simulink model "SEM_Battery"  (R2024a)
settings: Solver=FixedStepAuto  StartTime=0.0  StopTime=10.0  FixedStep=0.1  RelTol=1e-3
libraries: batteryecm_lib x96, fl_lib x4, nesl_utility x4, autolibmappedmotor x1
settings Model: Creator=v2578048  LastModifiedBy=marcelkaminski
settings RTWCC: GPUComputeCapability=3.5

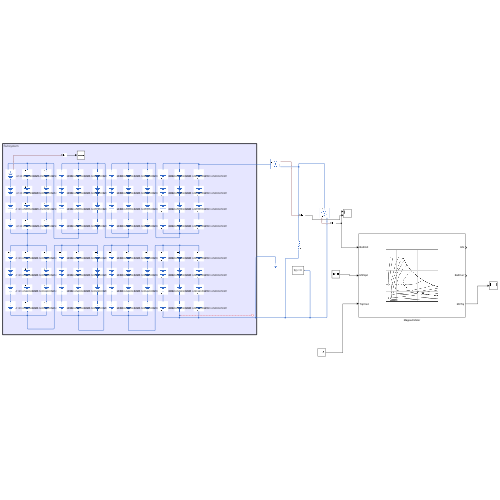
[thumbnail: Simulink's stored preview of the top-level diagram]
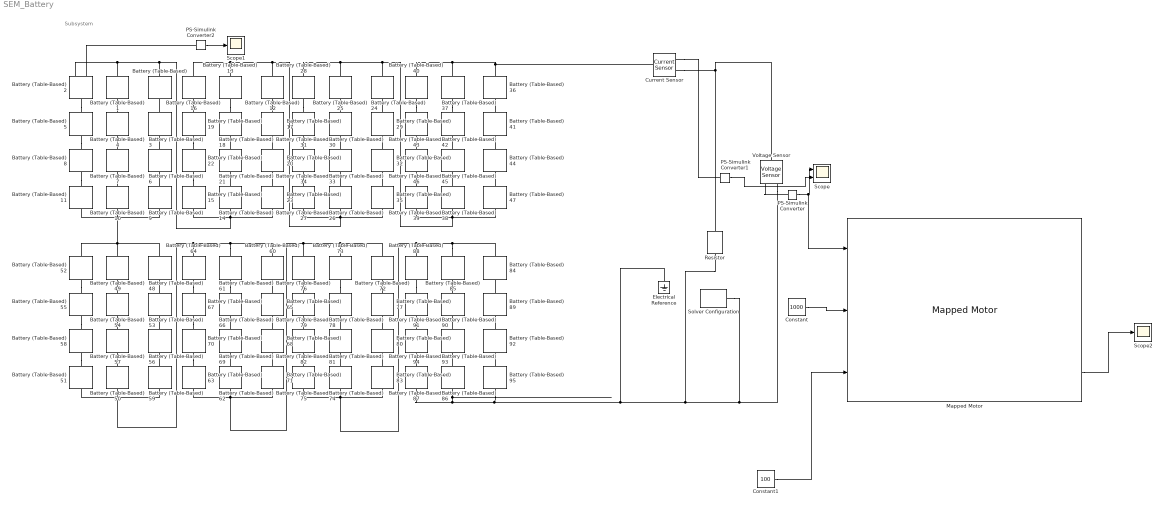
== system SEM_Battery ==
  note: Subsystem
  Battery (Table-Based){,1,3..95} (95 alike) : batteryecm_lib/Battery (Table-Based)  Tag={'toolbox/physmod/battery/shared_library/m/batteryecm_lib_parts';'Battery__Table_Based_/A123/ANR26650M1.xml'}  SOC_vec=[0 0.01 0.02 0.03 0.04 0.05 0.06 0.07 0.08 0.09 0.1 0.11 0.12 0.13 0.14 0.15 0.16 0.17 0.18 0.19 0.2 0.21 0.22 0.23 0.24 0.25 0.26 0.27 0.28 0.29 0.3 0.31 0.32 0.33 0.34 0.35 0.36 0.37 0.38 0.39 0.4 0.41 0.42 0.43 0.44 0.45 0.46 0.47 0.48 0.49 0.5 0.51 0.52 0.53 0.54 0.55 0.56 0.57 0.58 0.59 0.6 0.61 0.62 0.63 0.64 0.65 0.66 0.67 0.68 0.69 0.7 0.71 0.72 0.73 0.74 0.75 0.76 0.77 0.78 0.79 0.8 0.81 0.82 0.83 0.84 0.85 0.86 0.87 0.88 0.89 0.9 0.91 0.92 0.93 0.94 0.95 0.96 0.97 0.98 0.99 1]  T_dependence=simscape.enum.tablebattery.temperature_dependence.yes  prm_dir=simscape.enum.tablebattery.prm_dir.noCurrentDirectionality  T_vec=[-20 0 25] degC  V0_mat=[2.06518 2.06518 2.06518;2.68276 2.68276 2.68276;2.83127 2.83127 2.83127;2.93006 2.93006 2.93006;3.00018 3.00018 3.00018;3.05444 3.05444 3.05444;3.098 3.098 3.098;3.13677 3.13677 3.13677;3.17233 3.17233 3.17233;3.19687 3.19687 3.19687;3.20429 3.20429 3.20429;3.20797 3.20797 3.20797;3.21084 3.21084 3.21084;3.21322 3.21322 3.21322;3.21517 3.21517 3.21517;3.22057 3.22057 3.22057;3.22301 3.22301 3.22301;3.22946 3.22946 3.22946;3.23827 3.23827 3.23827;3.24173 3.24173 3.24173;3.24488 3.24488 3.24488;3.24931 3.24931 3.24931;3.2535 3.2535 3.2535;3.25765 3.25765 3.25765;3.26117 3.26117 3.26117;3.26357 3.26357 3.26357;3.26578 3.26578 3.26578;3.26981 3.26981 3.26981;3.27407 3.27407 3.27407;3.27754 3.27754 3.27754;3.27963 3.27963 3.27963;3.28165 3.28165 3.28165;3.28353 3.28353 3.28353;3.28542 3.28542 3.28542;3.28715 3.28715 3.28715;3.28889 3.28889 3.28889;3.29062 3.29062 3.29062;3.29275 3.29275 3.29275;3.29575 3.29575 3.29575;3.29889 3.29889 3.29889;3.30203 3.30203 3.30203;3.3027 3.3027 3.3027;3.30283 3.30283 3.30283;3.30242 3.30242 3.30242;3.30201 3.30201 3.30201;3.30226 3.30226 3.30226;3.30369 3.30369 3.30369;3.30511 3.30511 3.30511;3.3066 3.3066 3.3066;3.30845 3.30845 3.30845;3.30961 3.30961 3.30961;3.31045 3.31045 3.31045;3.31128 3.31128 3.31128;3.31212 3.31212 3.31212;3.31294 3.31294 3.31294;3.31336 3.31336 3.31336;3.31432 3.31432 3.31432;3.31596 3.31596 3.31596;3.3176 3.3176 3.3176;3.31906 3.31906 3.31906;3.32016 3.32016 3.32016;3.32147 3.32147 3.32147;3.32313 3.32313 3.32313;3.32479 3.32479 3.32479;3.32699 3.32699 3.32699;3.32924 3.32924 3.32924;3.33149 3.33149 3.33149;3.33281 3.33281 3.33281;3.33327 3.33327 3.33327;3.33363 3.33363 3.33363;3.33398 3.33398 3.33398;3.33434 3.33434 3.33434;3.33558 3.33558 3.33558;3.33748 3.33748 3.33748;3.33946 3.33946 3.33946;3.34145 3.34145 3.34145;3.34404 3.34404 3.34404;3.34672 3.34672 3.34672;3.34941 3.34941 3.34941;3.35026 3.35026 3.35026;3.35086 3.35086 3.35086;3.35091 3.35091 3.35091;3.35083 3.35083 3.35083;3.35192 3.35192 3.35192;3.35429 3.35429 3.35429;3.3566 3.3566 3.3566;3.35958 3.35958 3.35958;3.36218 3.36218 3.36218;3.36335 3.36335 3.36335;3.36552 3.36552 3.36552;3.36994 3.36994 3.36994;3.3722 3.3722 3.3722;3.3731 3.3731 3.3731;3.37515 3.37515 3.37515;3.37949 3.37949 3.37949;3.38971 3.38971 3.38971;3.40199 3.40199 3.40199;3.42645 3.42645 3.42645;3.48039 3.48039 3.48039;3.63268 3.63268 3.63268;3.84587 3.84587 3.84587] V  V0_vec=[2.06518 2.68276 2.83127 2.93006 3.00018 3.05444 3.098 3.13677 3.17233 3.19687 3.20429 3.20797 3.21084 3.21322 3.21517 3.22057 3.22301 3.22946 3.23827 3.24173 3.24488 3.24931 3.2535 3.25765 3.26117 3.26357 3.26578 3.26981 3.27407 3.27754 3.27963 3.28165 3.28353 3.28542 3.28715 3.28889 3.29062 3.29275 3.29575 3.29889 3.30203 3.3027 3.30283 3.30242 3.30201 3.30226 3.30369 3.30511 3.3066 3.30845 3.30961 3.31045 3.31128 3.31212 3.31294 3.31336 3.31432 3.31596 3.3176 3.31906 3.32016 3.32147 3.32313 3.32479 3.32699 3.32924 3.33149 3.33281 3.33327 3.33363 3.33398 3.33434 3.33558 3.33748 3.33946 3.34145 3.34404 3.34672 3.34941 3.35026 3.35086 3.35091 3.35083 3.35192 3.35429 3.3566 3.35958 3.36218 3.36335 3.36552 3.36994 3.3722 3.3731 3.37515 3.37949 3.38971 3.40199 3.42645 3.48039 3.63268 3.84587] V  V_range=[1.8 Inf] V  R0_mat=[0.28791 0.39917 0.03594;0.53384 0.62959 0.04836;0.57583 0.56865 0.04765;0.59621 0.50771 0.04556;0.60411 0.44678 0.04266;0.60512 0.38584 0.03932;0.60148 0.35318 0.03569;0.59575 0.33243 0.03191;0.58863 0.31331 0.02805;0.57672 0.29803 0.02388;0.55737 0.27565 0.02036;0.53639 0.25442 0.01833;0.51511 0.23302 0.01708;0.50085 0.21733 0.01587;0.48831 0.20337 0.01474;0.47733 0.19108 0.01411;0.46518 0.17861 0.01378;0.45492 0.16789 0.01359;0.44686 0.15933 0.01333;0.43712 0.15091 0.01312;0.42864 0.14235 0.01302;0.42073 0.13523 0.01308;0.41279 0.13112 0.01313;0.40493 0.127 0.01318;0.39734 0.12273 0.01323;0.38927 0.11936 0.01327;0.38209 0.11591 0.01333;0.37585 0.11324 0.01346;0.36956 0.11236 0.0136;0.36284 0.11117 0.01363;0.35652 0.10939 0.01363;0.35104 0.10772 0.01362;0.34554 0.10751 0.01361;0.34017 0.1073 0.01363;0.33473 0.10703 0.01368;0.32958 0.10675 0.01374;0.32594 0.10584 0.01379;0.32247 0.10427 0.01385;0.31911 0.10309 0.01395;0.31579 0.10197 0.01407;0.31253 0.1013 0.01419;0.30825 0.10101 0.01424;0.30375 0.10049 0.01428;0.29928 0.09973 0.01426;0.29512 0.09897 0.01424;0.29126 0.09851 0.01424;0.28925 0.09882 0.01427;0.28727 0.09919 0.01431;0.28531 0.09959 0.01435;0.2831 0.09941 0.01443;0.2802 0.09868 0.0145;0.27716 0.09781 0.01456;0.27412 0.09713 0.01462;0.26933 0.09664 0.01468;0.26437 0.09613 0.01473;0.26155 0.09545 0.01474;0.26216 0.09509 0.01476;0.26306 0.09503 0.0148;0.26159 0.09497 0.01484;0.25849 0.09478 0.01488;0.25493 0.09441 0.0149;0.25109 0.09413 0.01492;0.24864 0.09443 0.01498;0.24734 0.09474 0.01504;0.24628 0.09481 0.01513;0.24523 0.09489 0.01523;0.24431 0.09498 0.01532;0.24301 0.09496 0.01539;0.24134 0.09492 0.01543;0.23962 0.09482 0.01545;0.23798 0.09473 0.01547;0.23639 0.09464 0.0155;0.2352 0.09494 0.01554;0.23428 0.09522 0.01561;0.23339 0.09501 0.01566;0.23251 0.0948 0.01572;0.23188 0.09479 0.0158;0.23129 0.09474 0.01589;0.23109 0.09468 0.01598;0.2301 0.09394 0.01601;0.229 0.09311 0.01605;0.22766 0.09205 0.01609;0.22633 0.09165 0.01612;0.22553 0.09189 0.01613;0.22529 0.09268 0.01616;0.22504 0.09302 0.01619;0.22516 0.09346 0.01618;0.22512 0.09375 0.01594;0.22445 0.09333 0.0156;0.22379 0.09334 0.01534;0.22383 0.09429 0.01512;0.22294 0.09419 0.01474;0.22121 0.0935 0.01431;0.21784 0.09272 0.01395;0.21547 0.09199 0.01345;0.21296 0.09382 0.01301;0.20996 0.09444 0.01263;0.20584 0.09405 0.01235;0.21023 0.09408 0.01272;0.21135 0.10392 0.01483;0.19733 0.12789 0.01454] Ohm  R0_vec=[0.03594 0.04836 0.04765 0.04556 0.04266 0.03932 0.03569 0.03191 0.02805 0.02388 0.02036 0.01833 0.01708 0.01587 0.01474 0.01411 0.01378 0.01359 0.01333 0.01312 0.01302 0.01308 0.01313 0.01318 0.01323 0.01327 0.01333 0.01346 0.0136 0.01363 0.01363 0.01362 0.01361 0.01363 0.01368 0.01374 0.01379 0.01385 0.01395 0.01407 0.01419 0.01424 0.01428 0.01426 0.01424 0.01424 0.01427 0.01431 0.01435 0.01443 0.0145 0.01456 0.01462 0.01468 0.01473 0.01474 0.01476 0.0148 0.01484 0.01488 0.0149 0.01492 0.01498 0.01504 0.01513 0.01523 0.01532 0.01539 0.01543 0.01545 0.01547 0.0155 0.01554 0.01561 0.01566 0.01572 0.0158 0.01589 0.01598 0.01601 0.01605 0.01609 0.01612 0.01613 0.01616 0.01619 0.01618 0.01594 0.0156 0.01534 0.01512 0.01474 0.01431 0.01395 0.01345 0.01301 0.01263 0.01235 0.01272 0.01483 0.01454] Ohm  R0_dis_mat=[.0117, .0085, .009; .011, .0085, .009; .0114, .0087, .0092; .0107, .0082, .0088; .0107, .0083, .0091; .0113, .0085, .0089; .0116, .0085, .0089] % Parameter not set Ohm  R0_dis_vec=[.0085, .0085, .0087, .0082, .0083, .0085, .0085] % Parameter not set Ohm  R0_ch_mat=[.0117, .0085, .009; .011, .0085, .009; .0114, .0087, .0092; .0107, .0082, .0088; .0107, .0083, .0091; .0113, .0085, .0089; .0116, .0085, .0089] % Parameter not set Ohm  R0_ch_vec=[.0085, .0085, .0087, .0082, .0083, .0085, .0085] % Parameter not set Ohm  AH=2.341 hr*A  prm_leak=simscape.enum.tablebattery.prm_leak.disabled  Rleak_vec=[8000, 7000, 6000] % Parameter not set Ohm  Rleak=7e3 % Parameter not set Ohm  extrapolation_option=simscape.enum.extrapolation.nearest  SOC_port=simscape.enum.tablebattery.enable.no  prm_dyn=simscape.enum.tablebattery.prm_dyn.off  R1_mat=[.0109, .0029, .0013; .0069, .0024, .0012; .0047, .0026, .0013; .0034, .0016, .001; .0033, .0023, .0014; .0033, .0018, .0011; .0028, .0017, .0011] % Parameter not set Ohm  R1_vec=[.0029, .0024, .0026, .0016, .0023, .0018, .0017] % Parameter not set Ohm  tau1_mat=[20, 36, 39; 31, 45, 39; 109, 105, 61; 36, 29, 26; 59, 77, 67; 40, 33, 29; 25, 39, 33] % Parameter not set s  tau1_vec=[36, 45, 105, 29, 77, 33, 39] % Parameter not set s  R2_mat=[.0109, .0029, .0013; .0069, .0024, .0012; .0047, .0026, .0013; .0034, .0016, .001; .0033, .0023, .0014; .0033, .0018, .0011; .0028, .0017, .0011] % Parameter not set Ohm  R2_vec=[.0029, .0024, .0026, .0016, .0023, .0018, .0017] % Parameter not set Ohm  tau2_mat=[20, 36, 39; 31, 45, 39; 109, 105, 61; 36, 29, 26; 59, 77, 67; 40, 33, 29; 25, 39, 33] % Parameter not set s  tau2_vec=[36, 45, 105, 29, 77, 33, 39] % Parameter not set s  R3_mat=[.0109, .0029, .0013; .0069, .0024, .0012; .0047, .0026, .0013; .0034, .0016, .001; .0033, .0023, .0014; .0033, .0018, .0011; .0028, .0017, .0011] % Parameter not set Ohm  R3_vec=[.0029, .0024, .0026, .0016, .0023, .0018, .0017] % Parameter not set Ohm  tau3_mat=[20, 36, 39; 31, 45, 39; 109, 105, 61; 36, 29, 26; 59, 77, 67; 40, 33, 29; 25, 39, 33] % Parameter not set s  tau3_vec=[36, 45, 105, 29, 77, 33, 39] % Parameter not set s  R4_mat=[.0109, .0029, .0013; .0069, .0024, .0012; .0047, .0026, .0013; .0034, .0016, .001; .0033, .0023, .0014; .0033, .0018, .0011; .0028, .0017, .0011] % Parameter not set Ohm  R4_vec=[.0029, .0024, .0026, .0016, .0023, .0018, .0017] % Parameter not set Ohm  tau4_mat=[20, 36, 39; 31, 45, 39; 109, 105, 61; 36, 29, 26; 59, 77, 67; 40, 33, 29; 25, 39, 33] % Parameter not set s  tau4_vec=[36, 45, 105, 29, 77, 33, 39] % Parameter not set s  R5_mat=[.0109, .0029, .0013; .0069, .0024, .0012; .0047, .0026, .0013; .0034, .0016, .001; .0033, .0023, .0014; .0033, .0018, .0011; .0028, .0017, .0011] % Parameter not set Ohm  R5_vec=[.0029, .0024, .0026, .0016, .0023, .0018, .0017] % Parameter not set Ohm  tau5_mat=[20, 36, 39; 31, 45, 39; 109, 105, 61; 36, 29, 26; 59, 77, 67; 40, 33, 29; 25, 39, 33] % Parameter not set s  tau5_vec=[36, 45, 105, 29, 77, 33, 39] % Parameter not set s  prm_fade=simscape.enum.tablebattery.prm_fade.tableN  N0=100 % Parameter not set  dV0=0 % Parameter not set  dR0=0 % Parameter not set  dAH=0 % Parameter not set  dRleak=0 % Parameter not set  dR1=0 % Parameter not set  dR2=0 % Parameter not set  dR3=0 % Parameter not set  dR4=0 % Parameter not set  dR5=0 % Parameter not set  N0vec=[1 12 23 34 45 56 67 78 89 100 111 122 133 144 155 166 177 188 199 210 221 232 243 254 265 276 287 298 309 320 331 342 353 364 375 386 397 408 419 430 441 452 463 474 485 496 507 518 529 540 551 562 573 584 595 606 617 628 639 650 661 672 683 694 705 716 727 738 749 760 771 782 793 804 815 826 837 848 859 870 881 892 903 914 925 936 947 958 969 980 991 1002]  Tfadevec=[298.15, 323.15] % Parameter not set K  dV0vec=[0 -2.002 -2.6261 -2.9216 -3.1236 -3.3257 -3.5223 -3.7133 -3.9044 -4.2968 -4.7603 -5.2239 -5.6645 -6.0494 -6.4343 -6.8192 -7.2041 -7.3674 -7.2786 -7.1898 -7.101 -7.1198 -7.4721 -7.8245 -8.1769 -8.5292 -8.8816 -9.2733 -9.5616 -9.7015 -9.8414 -9.9678 -10.0299 -10.0919 -10.154 -10.216 -10.2781 -10.3402 -10.4448 -10.5636 -10.6824 -10.8012 -10.9056 -10.9361 -10.9667 -10.9972 -11.0226 -11.0377 -11.0527 -11.0678 -11.0979 -11.1585 -11.2191 -11.2797 -11.3402 -11.3884 -11.4143 -11.4403 -11.4662 -11.4921 -11.5332 -11.5611 -11.5848 -11.6085 -11.6323 -11.6445 -11.6495 -11.6545 -11.6594 -11.6644 -11.6693 -11.6918 -11.7308 -11.7699 -11.8089 -11.848 -11.8797 -11.8797 -11.8797 -11.8797 -11.8872 -11.8994 -11.9116 -11.9238 -11.9426 -11.968 -11.9934 -12.0155 -12.0345 -12.0535 -12.0755 -12.0979]  dR0vec=[0 0 0 0 0 0 0 0 0 0 0 0 0 0 0 0 0 0 0 0 0 0 0 0 0 0 0 0 0 0 0 0 0 0 0 0 0 0 0 0 0 0 0 0 0 0 0 0 0 0 0 0 0 0 0 0 0 0 0 0 0 0 0 0 0 0 0 0 0 0 0 0 0 0 0 0 0 0 0 0 0 0 0 0 0 0 0 0 0 0 0 0] % Parameter assumed  dAHvec=[0 -0.361 -0.474 -0.527 -0.564 -0.6 -0.635 -0.67 -0.704 -0.775 -0.859 -0.942 -1.031 -1.128 -1.225 -1.322 -1.419 -1.461 -1.438 -1.416 -1.393 -1.398 -1.487 -1.576 -1.665 -1.754 -1.843 -1.942 -2.042 -2.141 -2.241 -2.331 -2.376 -2.42 -2.464 -2.508 -2.553 -2.597 -2.671 -2.756 -2.841 -2.926 -3 -3.048 -3.096 -3.144 -3.184 -3.208 -3.231 -3.255 -3.302 -3.398 -3.493 -3.588 -3.683 -3.759 -3.8 -3.841 -3.881 -3.922 -3.987 -4.061 -4.135 -4.21 -4.284 -4.323 -4.338 -4.354 -4.369 -4.385 -4.4 -4.47 -4.593 -4.715 -4.837 -4.96 -5.071 -5.071 -5.071 -5.071 -5.099 -5.145 -5.191 -5.237 -5.307 -5.403 -5.499 -5.582 -5.653 -5.725 -5.807 -5.892]  dRleakvec=[0, 0, 0] % Parameter not set  dR1vec=[0, 0, 0] % Parameter not set  dR2vec=[0, 0, 0] % Parameter not set  dR3vec=[0, 0, 0] % Parameter not set  dR4vec=[0, 0, 0] % Parameter not set  dR5vec=[0, 0, 0] % Parameter not set  dV0mat=[0, 0; 0, 0; 0, 0] % Parameter not set  dR0mat=[0, 0; 0, 0; 0, 0] % Parameter not set  dAHmat=[0, 0; 0, 0; 0, 0] % Parameter not set  dRleakmat=[0, 0; 0, 0; 0, 0] % Parameter not set  dR1mat=[0, 0; 0, 0; 0, 0] % Parameter not set  dR2mat=[0, 0; 0, 0; 0, 0] % Parameter not set  dR3mat=[0, 0; 0, 0; 0, 0] % Parameter not set  dR4mat=[0, 0; 0, 0; 0, 0] % Parameter not set  dR5mat=[0, 0; 0, 0; 0, 0] % Parameter not set  prm_age_modeling=simscape.enum.tablebattery.prm_age_modeling.equation  storage_dt_age_vec=[0] % Parameter not set d  storage_T_age_vec=[273] % Parameter not set K  prm_age_OCV=simscape.enum.tablebattery.prm_age_OCV.OCV  OCV_age=0.9 % Parameter not set  SOC_age=0.6 % Parameter not set  prm_age_resistance=simscape.enum.tablebattery.prm_age.disabled  OCV_scaling_age_resistance=2.2134e6 % Parameter not set  OCV_offset_age_resistance=1.632e6 % Parameter not set  temp_exp_age_resistance=0.515833569 % Parameter not set V  t_exp_age_resistance=0.75 % Parameter not set  T_age_vec_resistance=[273.15, 298.15, 323.15] % Parameter not set K  dt_age_vec_resistance=[90, 180, 270, 360] % Parameter not set d  dR0_age_vec=[0, 0, 0] % Parameter not set  t_meas_dR0_age=100 % Parameter not set d  dR0_age_mat=[0, 0, 0; 0, 0, 0; 0, 0, 0; 0, 0, 0] % Parameter not set  prm_age_capacity=simscape.enum.tablebattery.prm_age.disabled  OCV_scaling_age_capacity=1.5097e07 % Parameter not set  OCV_offset_age_capacity=8.3625e06 % Parameter not set  temp_exp_age_capacity=0.6011 % Parameter not set V  t_exp_age_capacity=0.75 % Parameter not set  T_age_vec_capacity=[273.15, 298.15, 323.15] % Parameter not set K  dt_age_vec_capacity=[90, 180, 270, 360] % Parameter not set d  dAH_age_vec=[0, 0, 0] % Parameter not set  t_meas_dAH_age=100 % Parameter not set d  dAH_age_mat=[0, 0, 0; 0, 0, 0; 0, 0, 0; 0, 0, 0] % Parameter not set  thermal_port=simscape.enum.thermaleffects.omit  temperature=298.15 % Parameter not set K  thermal_mass=64.8 % Parameter assumed J/K  i_specify=off  i_priority=None  i=0 A  i_nominal_specify=off  i_nominal_value=1  i_nominal_unit=A  v_specify=off  v_priority=None  v=0 V  v_nominal_specify=off  v_nominal_value=1  v_nominal_unit=V  stateOfCharge_specify=off  stateOfCharge_priority=High  stateOfCharge=1  stateOfCharge_nominal_specify=off  stateOfCharge_nominal_value=1  stateOfCharge_nominal_unit=1  num_cycles_specify=off  num_cycles_priority=High  num_cycles=0  num_cycles_nominal_specify=off  num_cycles_nominal_value=1  num_cycles_nominal_unit=1  cell_temperature_specify=off  cell_temperature_priority=High  cell_temperature=298.15 K  cell_temperature_nominal_specify=off  cell_temperature_nominal_value=1  cell_temperature_nominal_unit=K
      settings: AttributesFormatString=A123:ANR26650M1  InternalSimscapePortConfiguration="{\"Bottom\":[],\"Left\":[{\"id\":\"p\",\"label\":\"+\",\"type\":\"foundation.electrical.electrical\"}],\"Right\":[{\"id\":\"n\",\"label\":\"-\",\"type\":\"foundation.electrical.electrical\"}],\"Top\":[]}"
      settings: LibrarySourceBlock=|
      | batt_lib/Cells/Battery
      | (Table-Based)
  Battery (Table-Based)2 : batteryecm_lib/Battery (Table-Based)  Tag={'toolbox/physmod/battery/shared_library/m/batteryecm_lib_parts';'Battery__Table_Based_/A123/ANR26650M1.xml'}  SOC_vec=[0 0.01 0.02 0.03 0.04 0.05 0.06 0.07 0.08 0.09 0.1 0.11 0.12 0.13 0.14 0.15 0.16 0.17 0.18 0.19 0.2 0.21 0.22 0.23 0.24 0.25 0.26 0.27 0.28 0.29 0.3 0.31 0.32 0.33 0.34 0.35 0.36 0.37 0.38 0.39 0.4 0.41 0.42 0.43 0.44 0.45 0.46 0.47 0.48 0.49 0.5 0.51 0.52 0.53 0.54 0.55 0.56 0.57 0.58 0.59 0.6 0.61 0.62 0.63 0.64 0.65 0.66 0.67 0.68 0.69 0.7 0.71 0.72 0.73 0.74 0.75 0.76 0.77 0.78 0.79 0.8 0.81 0.82 0.83 0.84 0.85 0.86 0.87 0.88 0.89 0.9 0.91 0.92 0.93 0.94 0.95 0.96 0.97 0.98 0.99 1]  T_dependence=simscape.enum.tablebattery.temperature_dependence.yes  prm_dir=simscape.enum.tablebattery.prm_dir.noCurrentDirectionality  T_vec=[-20 0 25] degC  V0_mat=[2.06518 2.06518 2.06518;2.68276 2.68276 2.68276;2.83127 2.83127 2.83127;2.93006 2.93006 2.93006;3.00018 3.00018 3.00018;3.05444 3.05444 3.05444;3.098 3.098 3.098;3.13677 3.13677 3.13677;3.17233 3.17233 3.17233;3.19687 3.19687 3.19687;3.20429 3.20429 3.20429;3.20797 3.20797 3.20797;3.21084 3.21084 3.21084;3.21322 3.21322 3.21322;3.21517 3.21517 3.21517;3.22057 3.22057 3.22057;3.22301 3.22301 3.22301;3.22946 3.22946 3.22946;3.23827 3.23827 3.23827;3.24173 3.24173 3.24173;3.24488 3.24488 3.24488;3.24931 3.24931 3.24931;3.2535 3.2535 3.2535;3.25765 3.25765 3.25765;3.26117 3.26117 3.26117;3.26357 3.26357 3.26357;3.26578 3.26578 3.26578;3.26981 3.26981 3.26981;3.27407 3.27407 3.27407;3.27754 3.27754 3.27754;3.27963 3.27963 3.27963;3.28165 3.28165 3.28165;3.28353 3.28353 3.28353;3.28542 3.28542 3.28542;3.28715 3.28715 3.28715;3.28889 3.28889 3.28889;3.29062 3.29062 3.29062;3.29275 3.29275 3.29275;3.29575 3.29575 3.29575;3.29889 3.29889 3.29889;3.30203 3.30203 3.30203;3.3027 3.3027 3.3027;3.30283 3.30283 3.30283;3.30242 3.30242 3.30242;3.30201 3.30201 3.30201;3.30226 3.30226 3.30226;3.30369 3.30369 3.30369;3.30511 3.30511 3.30511;3.3066 3.3066 3.3066;3.30845 3.30845 3.30845;3.30961 3.30961 3.30961;3.31045 3.31045 3.31045;3.31128 3.31128 3.31128;3.31212 3.31212 3.31212;3.31294 3.31294 3.31294;3.31336 3.31336 3.31336;3.31432 3.31432 3.31432;3.31596 3.31596 3.31596;3.3176 3.3176 3.3176;3.31906 3.31906 3.31906;3.32016 3.32016 3.32016;3.32147 3.32147 3.32147;3.32313 3.32313 3.32313;3.32479 3.32479 3.32479;3.32699 3.32699 3.32699;3.32924 3.32924 3.32924;3.33149 3.33149 3.33149;3.33281 3.33281 3.33281;3.33327 3.33327 3.33327;3.33363 3.33363 3.33363;3.33398 3.33398 3.33398;3.33434 3.33434 3.33434;3.33558 3.33558 3.33558;3.33748 3.33748 3.33748;3.33946 3.33946 3.33946;3.34145 3.34145 3.34145;3.34404 3.34404 3.34404;3.34672 3.34672 3.34672;3.34941 3.34941 3.34941;3.35026 3.35026 3.35026;3.35086 3.35086 3.35086;3.35091 3.35091 3.35091;3.35083 3.35083 3.35083;3.35192 3.35192 3.35192;3.35429 3.35429 3.35429;3.3566 3.3566 3.3566;3.35958 3.35958 3.35958;3.36218 3.36218 3.36218;3.36335 3.36335 3.36335;3.36552 3.36552 3.36552;3.36994 3.36994 3.36994;3.3722 3.3722 3.3722;3.3731 3.3731 3.3731;3.37515 3.37515 3.37515;3.37949 3.37949 3.37949;3.38971 3.38971 3.38971;3.40199 3.40199 3.40199;3.42645 3.42645 3.42645;3.48039 3.48039 3.48039;3.63268 3.63268 3.63268;3.84587 3.84587 3.84587] V  V0_vec=[2.06518 2.68276 2.83127 2.93006 3.00018 3.05444 3.098 3.13677 3.17233 3.19687 3.20429 3.20797 3.21084 3.21322 3.21517 3.22057 3.22301 3.22946 3.23827 3.24173 3.24488 3.24931 3.2535 3.25765 3.26117 3.26357 3.26578 3.26981 3.27407 3.27754 3.27963 3.28165 3.28353 3.28542 3.28715 3.28889 3.29062 3.29275 3.29575 3.29889 3.30203 3.3027 3.30283 3.30242 3.30201 3.30226 3.30369 3.30511 3.3066 3.30845 3.30961 3.31045 3.31128 3.31212 3.31294 3.31336 3.31432 3.31596 3.3176 3.31906 3.32016 3.32147 3.32313 3.32479 3.32699 3.32924 3.33149 3.33281 3.33327 3.33363 3.33398 3.33434 3.33558 3.33748 3.33946 3.34145 3.34404 3.34672 3.34941 3.35026 3.35086 3.35091 3.35083 3.35192 3.35429 3.3566 3.35958 3.36218 3.36335 3.36552 3.36994 3.3722 3.3731 3.37515 3.37949 3.38971 3.40199 3.42645 3.48039 3.63268 3.84587] V  V_range=[1.8 Inf] V  R0_mat=[0.28791 0.39917 0.03594;0.53384 0.62959 0.04836;0.57583 0.56865 0.04765;0.59621 0.50771 0.04556;0.60411 0.44678 0.04266;0.60512 0.38584 0.03932;0.60148 0.35318 0.03569;0.59575 0.33243 0.03191;0.58863 0.31331 0.02805;0.57672 0.29803 0.02388;0.55737 0.27565 0.02036;0.53639 0.25442 0.01833;0.51511 0.23302 0.01708;0.50085 0.21733 0.01587;0.48831 0.20337 0.01474;0.47733 0.19108 0.01411;0.46518 0.17861 0.01378;0.45492 0.16789 0.01359;0.44686 0.15933 0.01333;0.43712 0.15091 0.01312;0.42864 0.14235 0.01302;0.42073 0.13523 0.01308;0.41279 0.13112 0.01313;0.40493 0.127 0.01318;0.39734 0.12273 0.01323;0.38927 0.11936 0.01327;0.38209 0.11591 0.01333;0.37585 0.11324 0.01346;0.36956 0.11236 0.0136;0.36284 0.11117 0.01363;0.35652 0.10939 0.01363;0.35104 0.10772 0.01362;0.34554 0.10751 0.01361;0.34017 0.1073 0.01363;0.33473 0.10703 0.01368;0.32958 0.10675 0.01374;0.32594 0.10584 0.01379;0.32247 0.10427 0.01385;0.31911 0.10309 0.01395;0.31579 0.10197 0.01407;0.31253 0.1013 0.01419;0.30825 0.10101 0.01424;0.30375 0.10049 0.01428;0.29928 0.09973 0.01426;0.29512 0.09897 0.01424;0.29126 0.09851 0.01424;0.28925 0.09882 0.01427;0.28727 0.09919 0.01431;0.28531 0.09959 0.01435;0.2831 0.09941 0.01443;0.2802 0.09868 0.0145;0.27716 0.09781 0.01456;0.27412 0.09713 0.01462;0.26933 0.09664 0.01468;0.26437 0.09613 0.01473;0.26155 0.09545 0.01474;0.26216 0.09509 0.01476;0.26306 0.09503 0.0148;0.26159 0.09497 0.01484;0.25849 0.09478 0.01488;0.25493 0.09441 0.0149;0.25109 0.09413 0.01492;0.24864 0.09443 0.01498;0.24734 0.09474 0.01504;0.24628 0.09481 0.01513;0.24523 0.09489 0.01523;0.24431 0.09498 0.01532;0.24301 0.09496 0.01539;0.24134 0.09492 0.01543;0.23962 0.09482 0.01545;0.23798 0.09473 0.01547;0.23639 0.09464 0.0155;0.2352 0.09494 0.01554;0.23428 0.09522 0.01561;0.23339 0.09501 0.01566;0.23251 0.0948 0.01572;0.23188 0.09479 0.0158;0.23129 0.09474 0.01589;0.23109 0.09468 0.01598;0.2301 0.09394 0.01601;0.229 0.09311 0.01605;0.22766 0.09205 0.01609;0.22633 0.09165 0.01612;0.22553 0.09189 0.01613;0.22529 0.09268 0.01616;0.22504 0.09302 0.01619;0.22516 0.09346 0.01618;0.22512 0.09375 0.01594;0.22445 0.09333 0.0156;0.22379 0.09334 0.01534;0.22383 0.09429 0.01512;0.22294 0.09419 0.01474;0.22121 0.0935 0.01431;0.21784 0.09272 0.01395;0.21547 0.09199 0.01345;0.21296 0.09382 0.01301;0.20996 0.09444 0.01263;0.20584 0.09405 0.01235;0.21023 0.09408 0.01272;0.21135 0.10392 0.01483;0.19733 0.12789 0.01454] Ohm  R0_vec=[0.03594 0.04836 0.04765 0.04556 0.04266 0.03932 0.03569 0.03191 0.02805 0.02388 0.02036 0.01833 0.01708 0.01587 0.01474 0.01411 0.01378 0.01359 0.01333 0.01312 0.01302 0.01308 0.01313 0.01318 0.01323 0.01327 0.01333 0.01346 0.0136 0.01363 0.01363 0.01362 0.01361 0.01363 0.01368 0.01374 0.01379 0.01385 0.01395 0.01407 0.01419 0.01424 0.01428 0.01426 0.01424 0.01424 0.01427 0.01431 0.01435 0.01443 0.0145 0.01456 0.01462 0.01468 0.01473 0.01474 0.01476 0.0148 0.01484 0.01488 0.0149 0.01492 0.01498 0.01504 0.01513 0.01523 0.01532 0.01539 0.01543 0.01545 0.01547 0.0155 0.01554 0.01561 0.01566 0.01572 0.0158 0.01589 0.01598 0.01601 0.01605 0.01609 0.01612 0.01613 0.01616 0.01619 0.01618 0.01594 0.0156 0.01534 0.01512 0.01474 0.01431 0.01395 0.01345 0.01301 0.01263 0.01235 0.01272 0.01483 0.01454] Ohm  R0_dis_mat=[.0117, .0085, .009; .011, .0085, .009; .0114, .0087, .0092; .0107, .0082, .0088; .0107, .0083, .0091; .0113, .0085, .0089; .0116, .0085, .0089] % Parameter not set Ohm  R0_dis_vec=[.0085, .0085, .0087, .0082, .0083, .0085, .0085] % Parameter not set Ohm  R0_ch_mat=[.0117, .0085, .009; .011, .0085, .009; .0114, .0087, .0092; .0107, .0082, .0088; .0107, .0083, .0091; .0113, .0085, .0089; .0116, .0085, .0089] % Parameter not set Ohm  R0_ch_vec=[.0085, .0085, .0087, .0082, .0083, .0085, .0085] % Parameter not set Ohm  AH=2.341 hr*A  prm_leak=simscape.enum.tablebattery.prm_leak.disabled  Rleak_vec=[8000, 7000, 6000] % Parameter not set Ohm  Rleak=7e3 % Parameter not set Ohm  extrapolation_option=simscape.enum.extrapolation.nearest  SOC_port=simscape.enum.tablebattery.enable.yes  prm_dyn=simscape.enum.tablebattery.prm_dyn.off  R1_mat=[.0109, .0029, .0013; .0069, .0024, .0012; .0047, .0026, .0013; .0034, .0016, .001; .0033, .0023, .0014; .0033, .0018, .0011; .0028, .0017, .0011] % Parameter not set Ohm  R1_vec=[.0029, .0024, .0026, .0016, .0023, .0018, .0017] % Parameter not set Ohm  tau1_mat=[20, 36, 39; 31, 45, 39; 109, 105, 61; 36, 29, 26; 59, 77, 67; 40, 33, 29; 25, 39, 33] % Parameter not set s  tau1_vec=[36, 45, 105, 29, 77, 33, 39] % Parameter not set s  R2_mat=[.0109, .0029, .0013; .0069, .0024, .0012; .0047, .0026, .0013; .0034, .0016, .001; .0033, .0023, .0014; .0033, .0018, .0011; .0028, .0017, .0011] % Parameter not set Ohm  R2_vec=[.0029, .0024, .0026, .0016, .0023, .0018, .0017] % Parameter not set Ohm  tau2_mat=[20, 36, 39; 31, 45, 39; 109, 105, 61; 36, 29, 26; 59, 77, 67; 40, 33, 29; 25, 39, 33] % Parameter not set s  tau2_vec=[36, 45, 105, 29, 77, 33, 39] % Parameter not set s  R3_mat=[.0109, .0029, .0013; .0069, .0024, .0012; .0047, .0026, .0013; .0034, .0016, .001; .0033, .0023, .0014; .0033, .0018, .0011; .0028, .0017, .0011] % Parameter not set Ohm  R3_vec=[.0029, .0024, .0026, .0016, .0023, .0018, .0017] % Parameter not set Ohm  tau3_mat=[20, 36, 39; 31, 45, 39; 109, 105, 61; 36, 29, 26; 59, 77, 67; 40, 33, 29; 25, 39, 33] % Parameter not set s  tau3_vec=[36, 45, 105, 29, 77, 33, 39] % Parameter not set s  R4_mat=[.0109, .0029, .0013; .0069, .0024, .0012; .0047, .0026, .0013; .0034, .0016, .001; .0033, .0023, .0014; .0033, .0018, .0011; .0028, .0017, .0011] % Parameter not set Ohm  R4_vec=[.0029, .0024, .0026, .0016, .0023, .0018, .0017] % Parameter not set Ohm  tau4_mat=[20, 36, 39; 31, 45, 39; 109, 105, 61; 36, 29, 26; 59, 77, 67; 40, 33, 29; 25, 39, 33] % Parameter not set s  tau4_vec=[36, 45, 105, 29, 77, 33, 39] % Parameter not set s  R5_mat=[.0109, .0029, .0013; .0069, .0024, .0012; .0047, .0026, .0013; .0034, .0016, .001; .0033, .0023, .0014; .0033, .0018, .0011; .0028, .0017, .0011] % Parameter not set Ohm  R5_vec=[.0029, .0024, .0026, .0016, .0023, .0018, .0017] % Parameter not set Ohm  tau5_mat=[20, 36, 39; 31, 45, 39; 109, 105, 61; 36, 29, 26; 59, 77, 67; 40, 33, 29; 25, 39, 33] % Parameter not set s  tau5_vec=[36, 45, 105, 29, 77, 33, 39] % Parameter not set s  prm_fade=simscape.enum.tablebattery.prm_fade.tableN  N0=100 % Parameter not set  dV0=0 % Parameter not set  dR0=0 % Parameter not set  dAH=0 % Parameter not set  dRleak=0 % Parameter not set  dR1=0 % Parameter not set  dR2=0 % Parameter not set  dR3=0 % Parameter not set  dR4=0 % Parameter not set  dR5=0 % Parameter not set  N0vec=[1 12 23 34 45 56 67 78 89 100 111 122 133 144 155 166 177 188 199 210 221 232 243 254 265 276 287 298 309 320 331 342 353 364 375 386 397 408 419 430 441 452 463 474 485 496 507 518 529 540 551 562 573 584 595 606 617 628 639 650 661 672 683 694 705 716 727 738 749 760 771 782 793 804 815 826 837 848 859 870 881 892 903 914 925 936 947 958 969 980 991 1002]  Tfadevec=[298.15, 323.15] % Parameter not set K  dV0vec=[0 -2.002 -2.6261 -2.9216 -3.1236 -3.3257 -3.5223 -3.7133 -3.9044 -4.2968 -4.7603 -5.2239 -5.6645 -6.0494 -6.4343 -6.8192 -7.2041 -7.3674 -7.2786 -7.1898 -7.101 -7.1198 -7.4721 -7.8245 -8.1769 -8.5292 -8.8816 -9.2733 -9.5616 -9.7015 -9.8414 -9.9678 -10.0299 -10.0919 -10.154 -10.216 -10.2781 -10.3402 -10.4448 -10.5636 -10.6824 -10.8012 -10.9056 -10.9361 -10.9667 -10.9972 -11.0226 -11.0377 -11.0527 -11.0678 -11.0979 -11.1585 -11.2191 -11.2797 -11.3402 -11.3884 -11.4143 -11.4403 -11.4662 -11.4921 -11.5332 -11.5611 -11.5848 -11.6085 -11.6323 -11.6445 -11.6495 -11.6545 -11.6594 -11.6644 -11.6693 -11.6918 -11.7308 -11.7699 -11.8089 -11.848 -11.8797 -11.8797 -11.8797 -11.8797 -11.8872 -11.8994 -11.9116 -11.9238 -11.9426 -11.968 -11.9934 -12.0155 -12.0345 -12.0535 -12.0755 -12.0979]  dR0vec=[0 0 0 0 0 0 0 0 0 0 0 0 0 0 0 0 0 0 0 0 0 0 0 0 0 0 0 0 0 0 0 0 0 0 0 0 0 0 0 0 0 0 0 0 0 0 0 0 0 0 0 0 0 0 0 0 0 0 0 0 0 0 0 0 0 0 0 0 0 0 0 0 0 0 0 0 0 0 0 0 0 0 0 0 0 0 0 0 0 0 0 0] % Parameter assumed  dAHvec=[0 -0.361 -0.474 -0.527 -0.564 -0.6 -0.635 -0.67 -0.704 -0.775 -0.859 -0.942 -1.031 -1.128 -1.225 -1.322 -1.419 -1.461 -1.438 -1.416 -1.393 -1.398 -1.487 -1.576 -1.665 -1.754 -1.843 -1.942 -2.042 -2.141 -2.241 -2.331 -2.376 -2.42 -2.464 -2.508 -2.553 -2.597 -2.671 -2.756 -2.841 -2.926 -3 -3.048 -3.096 -3.144 -3.184 -3.208 -3.231 -3.255 -3.302 -3.398 -3.493 -3.588 -3.683 -3.759 -3.8 -3.841 -3.881 -3.922 -3.987 -4.061 -4.135 -4.21 -4.284 -4.323 -4.338 -4.354 -4.369 -4.385 -4.4 -4.47 -4.593 -4.715 -4.837 -4.96 -5.071 -5.071 -5.071 -5.071 -5.099 -5.145 -5.191 -5.237 -5.307 -5.403 -5.499 -5.582 -5.653 -5.725 -5.807 -5.892]  dRleakvec=[0, 0, 0] % Parameter not set  dR1vec=[0, 0, 0] % Parameter not set  dR2vec=[0, 0, 0] % Parameter not set  dR3vec=[0, 0, 0] % Parameter not set  dR4vec=[0, 0, 0] % Parameter not set  dR5vec=[0, 0, 0] % Parameter not set  dV0mat=[0, 0; 0, 0; 0, 0] % Parameter not set  dR0mat=[0, 0; 0, 0; 0, 0] % Parameter not set  dAHmat=[0, 0; 0, 0; 0, 0] % Parameter not set  dRleakmat=[0, 0; 0, 0; 0, 0] % Parameter not set  dR1mat=[0, 0; 0, 0; 0, 0] % Parameter not set  dR2mat=[0, 0; 0, 0; 0, 0] % Parameter not set  dR3mat=[0, 0; 0, 0; 0, 0] % Parameter not set  dR4mat=[0, 0; 0, 0; 0, 0] % Parameter not set  dR5mat=[0, 0; 0, 0; 0, 0] % Parameter not set  prm_age_modeling=simscape.enum.tablebattery.prm_age_modeling.equation  storage_dt_age_vec=[0] % Parameter not set d  storage_T_age_vec=[273] % Parameter not set K  prm_age_OCV=simscape.enum.tablebattery.prm_age_OCV.OCV  OCV_age=0.9 % Parameter not set  SOC_age=0.6 % Parameter not set  prm_age_resistance=simscape.enum.tablebattery.prm_age.disabled  OCV_scaling_age_resistance=2.2134e6 % Parameter not set  OCV_offset_age_resistance=1.632e6 % Parameter not set  temp_exp_age_resistance=0.515833569 % Parameter not set V  t_exp_age_resistance=0.75 % Parameter not set  T_age_vec_resistance=[273.15, 298.15, 323.15] % Parameter not set K  dt_age_vec_resistance=[90, 180, 270, 360] % Parameter not set d  dR0_age_vec=[0, 0, 0] % Parameter not set  t_meas_dR0_age=100 % Parameter not set d  dR0_age_mat=[0, 0, 0; 0, 0, 0; 0, 0, 0; 0, 0, 0] % Parameter not set  prm_age_capacity=simscape.enum.tablebattery.prm_age.disabled  OCV_scaling_age_capacity=1.5097e07 % Parameter not set  OCV_offset_age_capacity=8.3625e06 % Parameter not set  temp_exp_age_capacity=0.6011 % Parameter not set V  t_exp_age_capacity=0.75 % Parameter not set  T_age_vec_capacity=[273.15, 298.15, 323.15] % Parameter not set K  dt_age_vec_capacity=[90, 180, 270, 360] % Parameter not set d  dAH_age_vec=[0, 0, 0] % Parameter not set  t_meas_dAH_age=100 % Parameter not set d  dAH_age_mat=[0, 0, 0; 0, 0, 0; 0, 0, 0; 0, 0, 0] % Parameter not set  thermal_port=simscape.enum.thermaleffects.omit  temperature=298.15 % Parameter not set K  thermal_mass=64.8 % Parameter assumed J/K  i_specify=off  i_priority=None  i=0 A  i_nominal_specify=off  i_nominal_value=1  i_nominal_unit=A  v_specify=off  v_priority=None  v=0 V  v_nominal_specify=off  v_nominal_value=1  v_nominal_unit=V  stateOfCharge_specify=off  stateOfCharge_priority=High  stateOfCharge=1  stateOfCharge_nominal_specify=off  stateOfCharge_nominal_value=1  stateOfCharge_nominal_unit=1  num_cycles_specify=off  num_cycles_priority=High  num_cycles=0  num_cycles_nominal_specify=off  num_cycles_nominal_value=1  num_cycles_nominal_unit=1  cell_temperature_specify=off  cell_temperature_priority=High  cell_temperature=298.15 K  cell_temperature_nominal_specify=off  cell_temperature_nominal_value=1  cell_temperature_nominal_unit=K
      settings: AttributesFormatString=A123:ANR26650M1  InternalSimscapePortConfiguration="{\"Bottom\":[],\"Left\":[{\"id\":\"p\",\"label\":\"+\",\"type\":\"foundation.electrical.electrical\"},{\"id\":\"soc\",\"label\":\"SOC\",\"type\":\"output\"}],\"Right\":[{\"id\":\"n\",\"label\":\"-\",\"type\":\"foundation.electrical.electrical\"}],\"Top\":[]}"
      settings: LibrarySourceBlock=|
      | batt_lib/Cells/Battery
      | (Table-Based)
  Constant : Constant  Value=1000
  Constant1 : Constant  Value=100
  Current Sensor : fl_lib/Electrical/Electrical Sensors/Current Sensor
  Electrical Reference : fl_lib/Electrical/Electrical Elements/Electrical Reference
  Mapped Motor : autolibmappedmotor/Mapped Motor  port_config=Speed  param_by=Tabulated torque-speed envelope  w_t=[ 0 375 750 800 ]  T_t=[0.09 0.08 0.07 0]  torque_max=.1  power_max=30  Tc=0.02  param_loss=Single efficiency measurement  eff=100  w_eff=375  T_eff=0.08  Piron=0  Pbase=0  w_eff_bp=[-800 -400 0 400 800]  T_eff_bp=[0 0.03 0.06 0.09]  Temp_eff_bp=[233.15 293.15 373.15]  losses_table=[1.49 1.67 2.21 3.10; 0.42 0.69 1.14 2.03; 0.06 0.24 0.78 1.68; 0.42 0.69 1.14 2.03; 1.49 1.67 2.21 3.10]  losses_table_3d=cat(3,[1.49 1.67 2.21 3.10; 0.42 0.69 1.14 2.03; 0.06 0.24 0.78 1.68; 0.42 0.69 1.14 2.03; 1.49 1.67 2.21 3.10],[1.49 1.67 2.21 3.10; 0.42 0.69 1.14 2.03; 0.06 0.24 0.78 1.68; 0.42 0.69 1.14 2.03; 1.49 1.67 2.21 3.10],[1.49 1.67 2.21 3.10; 0.42 0.69 1.14 2.03; 0.06 0.24 0.78 1.68; 0.42 0.69 1.14 2.03; 1.49 1.67 2.21 3.10])  efficiency_table=[95 95 95 95; 95 95 95 95; 95 95 95 95; 95 95 95 95; 95 95 95 95]  efficiency_table_3d=cat(3,[95 95 95 95; 95 95 95 95; 95 95 95 95; 95 95 95 95; 95 95 95 95],[95 95 95 95; 95 95 95 95; 95 95 95 95; 95 95 95 95; 95 95 95 95],[95 95 95 95; 95 95 95 95; 95 95 95 95; 95 95 95 95; 95 95 95 95])  J=5e-6  b=1e-5  omega_o=0  T_t_extended=[0 0.07 0.08 0.09 0.08 0.07 0]  w_t_extended=[-800 -750 -375 0 375 750 800]  KLossIron=0  KLossCopper=0  x_w_eff_vec=[-8000 -4000 0 4000 8000]  x_T_eff_vec=[-0.09 -0.06 -0.03 0 0.03 0.06 0.09]  x_tmp_eff_vec=[-0.09 -0.06 -0.03 0 0.03 0.06 0.09]  x_losses_mat=[3.1 2.21 1.67 1.49 1.67 2.21 3.1;2.03 1.14 0.69 0.42 0.69 1.14 2.03;1.68 0.78 0.24 0.06 0.24 0.78 1.68;2.03 1.14 0.69 0.42 0.69 1.14 2.03;3.1 2.21 1.67 1.49 1.67 2.21 3.1]  x_losses_mat_3d=[37.8947368421052 25.2631578947368 12.6315789473684 0 12 24 36;18.9473684210526 12.6315789473684 6.3157894736842 0 5.99999999999999 12 18;0 0 0 0 0 0 0;18 12 5.99999999999999 0 6.3157894736842 12.6315789473684 18.9473684210526;36 24 12 0 12.6315789473684 25.2631578947368 37.8947368421052]  CalLossMapData={}  CalLossWithTempMapData={}  aMode=1  RefBlkName='autolibmappedmotor/Mapped Motor'
      settings: LibrarySourceBlock=autolibemachines/Mapped Motor
  PS-Simulink Converter : nesl_utility/PS-Simulink Converter  PhysicalDomain=network_engine_domain  SubClassName=ps_output  LeftPortType=input  RightPortType=output  PseudoPeriodic=off  Frequencies=[]  VectorFormat=inherit  Unit=inherit  AffineConversion=off
  PS-Simulink Converter1 : nesl_utility/PS-Simulink Converter  PhysicalDomain=network_engine_domain  SubClassName=ps_output  LeftPortType=input  RightPortType=output  PseudoPeriodic=off  Frequencies=[]  VectorFormat=inherit  Unit=inherit  AffineConversion=off
  PS-Simulink Converter2 : nesl_utility/PS-Simulink Converter  PhysicalDomain=network_engine_domain  SubClassName=ps_output  LeftPortType=input  RightPortType=output  PseudoPeriodic=off  Frequencies=[]  VectorFormat=inherit  Unit=inherit  AffineConversion=off
  Resistor : fl_lib/Electrical/Electrical Elements/Resistor  R=1 Ohm  i_specify=off  i_priority=None  i=0 A  i_nominal_specify=off  i_nominal_value=1  i_nominal_unit=A  v_specify=off  v_priority=None  v=0 V  v_nominal_specify=off  v_nominal_value=1  v_nominal_unit=V
  Scope : Scope  NumInputPorts=2
  Scope1 : Scope
  Scope2 : Scope
  Solver Configuration : nesl_utility/Solver Configuration  PhysicalDomain=network_engine_domain  SubClassName=solver  LeftPortType=input  RightPortType=generic  Tones=[]  Harmonics=[]  SimulateNoise=off  Profile=off  UseLocalSampling=off  EnableSwitchedLinearOptims=on  FrequencyDomain=off  UseCCode=off  RelTol=0.001  AbsTol=0.001  MinStep=1e-09  ToWorkspace=off  RevertToSquareIcSolve=off  NumHomotopyIterations=100  PhasorMode=off  PhasorModeNumHarmonics=1  ConsistencySolver=NEWTON_XTOL_AFTER_FTOL  IndexReductionMethod=DerivativeReplacement  DoDC=off  ResidualTolerance=1e-09  ConsistencyTolSource=GLOBAL  ConsistencyAbsTol=0.001  ConsistencyRelTol=0.001  ConsistencyTolFactor=0.001  UseLocalSolver=off  LocalSolverChoice=NE_BACKWARD_EULER_ADVANCER  ResolveIndetEquations=on  FunctionEvalNumThread=1  LocalSolverSampleTime=0.001  DoFixedCost=off  MaxNonlinIter=3  MaxModeIter=2  ComputeImpulses=off  ImpulseIterations=2  LinearAlgebra=auto  LinearAlgebraNumThread=0  EquationFormulation=NE_TIME_EF  DelaysMemoryBudget=1024  AutomaticFiltering=on  FilteringTimeConstant=0.001  PartitionStorageMethod=AS_NEEDED  PartitionMemoryBudget=1024  PartitionMethod=ROBUST  MultibodyUseLocalSolver=off  MultibodyLocalSolverChoice=ODE1  MultibodyLocalSolverSampleTime=0.001
  Voltage Sensor : fl_lib/Electrical/Electrical Sensors/Voltage Sensor
  wires:
  PS-Simulink Converter/1 -> Mapped Motor/1, Scope/1
  PS-Simulink Converter1/1 -> Scope/2
  PS-Simulink Converter2/1 -> Scope1/1
  Constant/1 -> Mapped Motor/2
  Constant1/1 -> Mapped Motor/3
  Mapped Motor/3 -> Scope2/1
  connections:
  PS-Simulink Converter/LConn1 -- Voltage Sensor/RConn1
  Current Sensor/RConn1 -- PS-Simulink Converter1/LConn1
  Battery (Table-Based)2/LConn2 -- PS-Simulink Converter2/LConn1
  Battery (Table-Based)94/RConn1 -- Battery (Table-Based)87/LConn1
  Battery (Table-Based)89/LConn1 -- Battery (Table-Based)84/RConn1
  Battery (Table-Based)95/LConn1 -- Battery (Table-Based)92/RConn1
  Battery (Table-Based)86/LConn1 -- Battery (Table-Based)93/RConn1
  Battery (Table-Based)85/RConn1 -- Battery (Table-Based)90/LConn1
  Battery (Table-Based)91/RConn1 -- Battery (Table-Based)94/LConn1
  Battery (Table-Based)92/LConn1 -- Battery (Table-Based)89/RConn1
  Battery (Table-Based)77/LConn1 -- Battery (Table-Based)72/RConn1
  Battery (Table-Based)83/LConn1 -- Battery (Table-Based)80/RConn1
  Battery (Table-Based)80/LConn1 -- Battery (Table-Based)77/RConn1
  Battery (Table-Based)74/LConn1 -- Battery (Table-Based)81/RConn1
  Battery (Table-Based)82/RConn1 -- Battery (Table-Based)75/LConn1
  Battery (Table-Based)73/RConn1 -- Battery (Table-Based)78/LConn1
  Battery (Table-Based)76/RConn1 -- Battery (Table-Based)79/LConn1
  Battery (Table-Based)62/LConn1 -- Battery (Table-Based)69/RConn1
  Battery (Table-Based)64/RConn1 -- Battery (Table-Based)67/LConn1
  Battery (Table-Based)67/RConn1 -- Battery (Table-Based)70/LConn1
  Battery (Table-Based)65/LConn1 -- Battery (Table-Based)60/RConn1
  Battery (Table-Based)49/RConn1 -- Battery (Table-Based)54/LConn1
  Solver Configuration/RConn1 -- Battery (Table-Based)86/RConn1 -- Battery (Table-Based)87/RConn1 -- Battery (Table-Based)95/RConn1 -- Electrical Reference/LConn1 -- Resistor/RConn1 -- Voltage Sensor/RConn2
  Battery (Table-Based)44/LConn1 -- Battery (Table-Based)41/RConn1
  Battery (Table-Based)33/LConn1 -- Battery (Table-Based)30/RConn1
  Battery (Table-Based)26/LConn1 -- Battery (Table-Based)33/RConn1
  Battery (Table-Based)46/RConn1 -- Battery (Table-Based)39/LConn1
  Battery (Table-Based)93/LConn1 -- Battery (Table-Based)90/RConn1
  Battery (Table-Based)59/LConn1 -- Battery (Table-Based)56/RConn1
  Battery (Table-Based)25/RConn1 -- Battery (Table-Based)30/LConn1
  Battery (Table-Based)29/LConn1 -- Battery (Table-Based)24/RConn1
  Battery (Table-Based)40/LConn1 -- Current Sensor/LConn1 -- Battery (Table-Based)36/LConn1 -- Battery (Table-Based)37/LConn1
  Battery (Table-Based)61/RConn1 -- Battery (Table-Based)66/LConn1
  Battery (Table-Based)69/LConn1 -- Battery (Table-Based)66/RConn1
  Battery (Table-Based)1/RConn1 -- Battery (Table-Based)4/LConn1
  Battery (Table-Based)52/RConn1 -- Battery (Table-Based)55/LConn1
  Battery (Table-Based)2/RConn1 -- Battery (Table-Based)5/LConn1
  Battery (Table-Based)57/LConn1 -- Battery (Table-Based)54/RConn1
  Battery (Table-Based)23/LConn1 -- Battery (Table-Based)20/RConn1
  Battery (Table-Based)85/LConn1 -- Battery (Table-Based)88/LConn1 -- Battery (Table-Based)75/RConn1 -- Battery (Table-Based)83/RConn1 -- Battery (Table-Based)74/RConn1 -- Battery (Table-Based)84/LConn1
  Battery (Table-Based)34/RConn1 -- Battery (Table-Based)27/LConn1
  Battery (Table-Based)58/RConn1 -- Battery (Table-Based)51/LConn1
  Battery (Table-Based)16/RConn1 -- Battery (Table-Based)19/LConn1
  Battery (Table-Based)81/LConn1 -- Battery (Table-Based)78/RConn1
  Battery (Table-Based)35/LConn1 -- Battery (Table-Based)32/RConn1
  Battery (Table-Based)14/LConn1 -- Battery (Table-Based)21/RConn1
  Battery (Table-Based)19/RConn1 -- Battery (Table-Based)22/LConn1
  Battery (Table-Based)45/LConn1 -- Battery (Table-Based)42/RConn1
  Battery (Table-Based)20/LConn1 -- Battery (Table-Based)17/RConn1
  Battery (Table-Based)22/RConn1 -- Battery (Table-Based)15/LConn1
  Battery (Table-Based)71/LConn1 -- Battery (Table-Based)68/RConn1
  Battery (Table-Based)37/RConn1 -- Battery (Table-Based)42/LConn1
  Battery (Table-Based)47/LConn1 -- Battery (Table-Based)44/RConn1
  Battery (Table-Based)28/RConn1 -- Battery (Table-Based)31/LConn1
  Battery (Table-Based)38/LConn1 -- Battery (Table-Based)45/RConn1
  Battery (Table-Based)55/RConn1 -- Battery (Table-Based)58/LConn1
  Battery (Table-Based)17/LConn1 -- Battery (Table-Based)12/RConn1
  Battery (Table-Based)53/LConn1 -- Battery (Table-Based)48/RConn1
  Battery (Table-Based)79/RConn1 -- Battery (Table-Based)82/LConn1
  Battery (Table-Based)70/RConn1 -- Battery (Table-Based)63/LConn1
  Battery (Table-Based)28/LConn1 -- Battery (Table-Based)24/LConn1 -- Battery (Table-Based)39/RConn1 -- Battery (Table-Based)47/RConn1 -- Battery (Table-Based)38/RConn1 -- Battery (Table-Based)25/LConn1
  Battery (Table-Based)7/LConn1 -- Battery (Table-Based)4/RConn1
  Battery (Table-Based)3/LConn1 -- Battery (Table-Based)/RConn1
  Battery (Table-Based)61/LConn1 -- Battery (Table-Based)64/LConn1 -- Battery (Table-Based)51/RConn1 -- Battery (Table-Based)59/RConn1 -- Battery (Table-Based)50/RConn1 -- Battery (Table-Based)60/LConn1
  Battery (Table-Based)50/LConn1 -- Battery (Table-Based)57/RConn1
  Battery (Table-Based)2/LConn1 -- Battery (Table-Based)/LConn1 -- Battery (Table-Based)15/RConn1 -- Battery (Table-Based)23/RConn1 -- Battery (Table-Based)14/RConn1 -- Battery (Table-Based)1/LConn1
  Battery (Table-Based)5/RConn1 -- Battery (Table-Based)8/LConn1
  Battery (Table-Based)32/LConn1 -- Battery (Table-Based)29/RConn1
  Battery (Table-Based)88/RConn1 -- Battery (Table-Based)91/LConn1
  Battery (Table-Based)56/LConn1 -- Battery (Table-Based)53/RConn1
  Battery (Table-Based)52/LConn1 -- Battery (Table-Based)49/LConn1 -- Battery (Table-Based)11/RConn1 -- Battery (Table-Based)9/RConn1 -- Battery (Table-Based)10/RConn1 -- Battery (Table-Based)48/LConn1
  Battery (Table-Based)43/RConn1 -- Battery (Table-Based)46/LConn1
  Battery (Table-Based)68/LConn1 -- Battery (Table-Based)65/RConn1
  Battery (Table-Based)73/LConn1 -- Battery (Table-Based)76/LConn1 -- Battery (Table-Based)63/RConn1 -- Battery (Table-Based)71/RConn1 -- Battery (Table-Based)62/RConn1 -- Battery (Table-Based)72/LConn1
  Battery (Table-Based)41/LConn1 -- Battery (Table-Based)36/RConn1
  Battery (Table-Based)6/LConn1 -- Battery (Table-Based)3/RConn1
  Battery (Table-Based)10/LConn1 -- Battery (Table-Based)7/RConn1
  Battery (Table-Based)40/RConn1 -- Battery (Table-Based)43/LConn1
  Battery (Table-Based)21/LConn1 -- Battery (Table-Based)18/RConn1
  Battery (Table-Based)8/RConn1 -- Battery (Table-Based)11/LConn1
  Battery (Table-Based)31/RConn1 -- Battery (Table-Based)34/LConn1
  Battery (Table-Based)16/LConn1 -- Battery (Table-Based)12/LConn1 -- Battery (Table-Based)27/RConn1 -- Battery (Table-Based)35/RConn1 -- Battery (Table-Based)26/RConn1 -- Battery (Table-Based)13/LConn1
  Battery (Table-Based)9/LConn1 -- Battery (Table-Based)6/RConn1
  Battery (Table-Based)13/RConn1 -- Battery (Table-Based)18/LConn1
  Voltage Sensor/LConn1 -- Current Sensor/RConn2 -- Resistor/LConn1
